simulink model "parkingNavigation_ErrorModel"  (R2021b)
settings: Solver=VariableStepAuto  StartTime=0.0  StopTime=1000  FixedStep=0.01  RelTol=1e-3
model workspace (MAT data in the model file):
  enableTransmit = 1
values from neighbouring files (symbols this model uses):
  accel_noise_deviation = 1e-3    (= 0.001)    [init.m]
  accel_scale_factor = 3e-6    (= 3e-06)    [init.m]
  accel_zero_offset = 5e-3    (= 0.005)    [init.m]
  alt_error_deviation = 1.5    [init.m]
  gyro_drift_const = deg2rad(0.02)/3600    [init.m]
  gyro_noise_deviation = deg2rad(0.01)/3600    [init.m]
  gyro_scale_factor = 5e-5    (= 5e-05)    [init.m]
  lat_error_deviation = 1.5    [init.m]
  lon_error_deviation = 1.5    [init.m]
  vel_e_error_deviation = 0.01    [init.m]
  vel_h_error_deviation = 0.01    [init.m]
  vel_n_error_deviation = 0.01    [init.m]
libraries: simulink x2
settings Model: Creator=Vladik  LastModifiedBy=Vladik

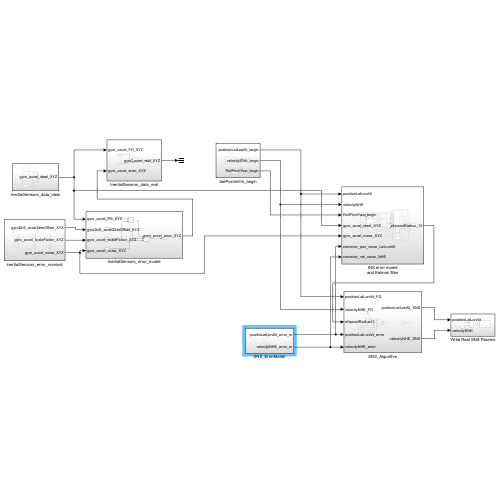
[thumbnail: Simulink's stored preview of the top-level diagram]
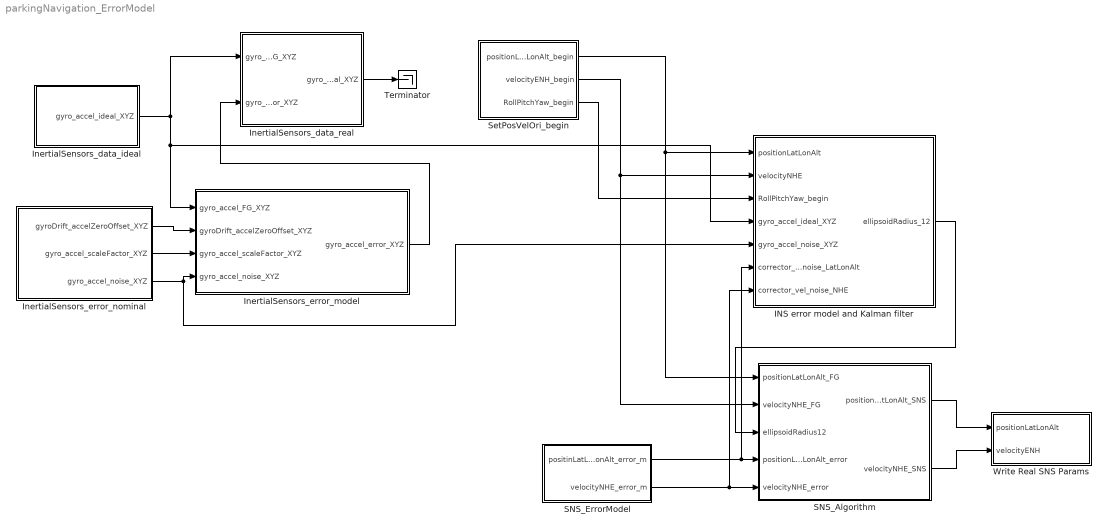
== system parkingNavigation_ErrorModel ==
  INS error model and Kalman filter : Subsystem
  InertialSensors_data_ideal : Subsystem
  InertialSensors_data_real : Subsystem
  InertialSensors_error_model : Subsystem
  InertialSensors_error_nominal : Subsystem
  SNS_Algorithm : Subsystem
  SNS_ErrorModel : Subsystem
  SetPosVelOri_begin : Subsystem
  Terminator : Terminator
  Write Real SNS Params : Subsystem
  wires:
  InertialSensors_data_ideal/1(gyro_accel_ideal_XYZ) -> InertialSensors_error_model/1(gyro_accel_FG_XYZ), INS error model and Kalman filter/4(gyro_accel_ideal_XYZ), InertialSensors_data_real/1(gyro_accel_FG_XYZ)
  InertialSensors_error_nominal/3(gyro_accel_noise_XYZ) -> InertialSensors_error_model/4(gyro_accel_noise_XYZ), INS error model and Kalman filter/5(gyro_accel_noise_XYZ)
  InertialSensors_error_nominal/2(gyro_accel_scaleFactor_XYZ) -> InertialSensors_error_model/3(gyro_accel_scaleFactor_XYZ)
  InertialSensors_error_nominal/1(gyroDrift_accelZeroOffset_XYZ) -> InertialSensors_error_model/2(gyroDrift_accelZeroOffset_XYZ)
  InertialSensors_error_model/1(gyro_accel_error_XYZ) -> InertialSensors_data_real/2(gyro_accel_error_XYZ)
  InertialSensors_data_real/1(gyro_accel_real_XYZ) -> Terminator/1
  SNS_ErrorModel/1(positinLatLonAlt_error_m) -> INS error model and Kalman filter/6(corrector_pos_noise_LatLonAlt), SNS_Algorithm/4(positionLatLonAlt_error)
  SNS_ErrorModel/2(velocityNHE_error_m) -> INS error model and Kalman filter/7(corrector_vel_noise_NHE), SNS_Algorithm/5(velocityNHE_error)
  SNS_Algorithm/1(positionLatLonAlt_SNS) -> Write Real SNS Params/1(positionLatLonAlt)
  SNS_Algorithm/2(velocityNHE_SNS) -> Write Real SNS Params/2(velocityENH)
  SetPosVelOri_begin/1(positionLatLonAlt_begin) -> INS error model and Kalman filter/1(positionLatLonAlt), SNS_Algorithm/1(positionLatLonAlt_FG)
  SetPosVelOri_begin/2(velocityENH_begin) -> INS error model and Kalman filter/2(velocityNHE), SNS_Algorithm/2(velocityNHE_FG)
  SetPosVelOri_begin/3(RollPitchYaw_begin) -> INS error model and Kalman filter/3(RollPitchYaw_begin)
  INS error model and Kalman filter/1(ellipsoidRadius_12) -> SNS_Algorithm/3(ellipsoidRadius12)

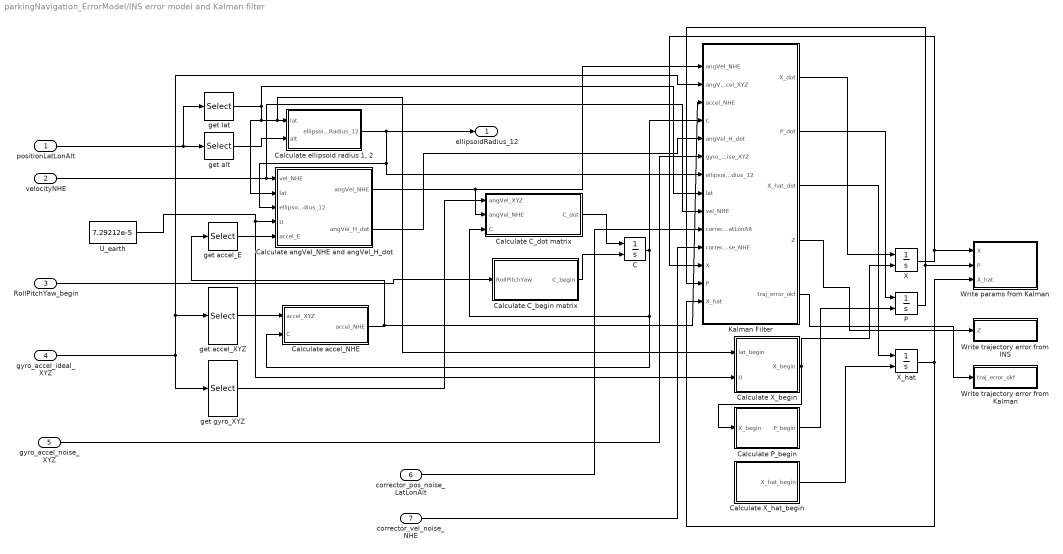
== system parkingNavigation_ErrorModel/INS error model and Kalman filter ==
  positionLatLonAlt : Inport
  velocityNHE : Inport  Port=2
  RollPitchYaw_begin : Inport  Port=3
  gyro_accel_ideal_XYZ : Inport  Port=4
  gyro_accel_noise_XYZ : Inport  Port=5
  corrector_pos_noise_LatLonAlt : Inport  Port=6
  corrector_vel_noise_NHE : Inport  Port=7
  C : Integrator  InitialConditionSource=external
  Calculate C_begin matrix : MATLAB Function  TreatAsAtomicUnit=on
  Calculate C_dot matrix : MATLAB Function  TreatAsAtomicUnit=on
  Calculate P_begin : MATLAB Function  TreatAsAtomicUnit=on
  Calculate X_begin : MATLAB Function  TreatAsAtomicUnit=on
  Calculate X_hat_begin : MATLAB Function  TreatAsAtomicUnit=on
  Calculate accel_NHE : MATLAB Function  TreatAsAtomicUnit=on
  Calculate angVel_NHE and angVel_H_dot : MATLAB Function  TreatAsAtomicUnit=on
  "Calculate ellipsoid radius 1, 2" : MATLAB Function  TreatAsAtomicUnit=on
  Kalman Filter : MATLAB Function  TreatAsAtomicUnit=on
  P : Integrator  InitialConditionSource=external
  U_earth : Constant  Value=7.29212e-5
  Write params from Kalman : Subsystem
  Write trajectory error from INS : Subsystem
  Write trajectory error from Kalman : Subsystem
  X : Integrator  InitialConditionSource=external
  X_hat : Integrator  InitialConditionSource=external
  get accel_E : Selector  InputPortWidth=3  IndexOptions=Index vector (dialog)  Indices=[3]  OutputSizes=1
  get accel_XYZ : Selector  InputPortWidth=6  IndexOptions=Index vector (dialog)  Indices=[4 5 6]  OutputSizes=1
  get alt : Selector  InputPortWidth=3  IndexOptions=Index vector (dialog)  Indices=[3]  OutputSizes=1
  get gyro_XYZ : Selector  InputPortWidth=6  IndexOptions=Index vector (dialog)  Indices=[1 2 3]  OutputSizes=1
  get lat : Selector  InputPortWidth=3  IndexOptions=Index vector (dialog)  Indices=[1]  OutputSizes=1
  ellipsoidRadius_12 : Outport
  wires:
  Kalman Filter/5(traj_error_okf) -> Write trajectory error from Kalman/1(traj_error_okf)
  corrector_vel_noise_NHE/1 -> Kalman Filter/11(corrector_vel_noise_NHE)
  gyro_accel_ideal_XYZ/1 -> get accel_XYZ/1, Kalman Filter/2(angVel_accel_XYZ), get gyro_XYZ/1
  get accel_XYZ/1 -> Calculate accel_NHE/1(accel_XYZ)
  get lat/1 -> Calculate angVel_NHE and angVel_H_dot/2(lat), Calculate X_begin/1(lat_begin), "Calculate ellipsoid radius 1, 2"/1(lat), Kalman Filter/8(lat)
  X/1 -> Write params from Kalman/1(X), Kalman Filter/12(X)
  Calculate C_begin matrix/1(C_begin) -> C/2
  C/1 -> Calculate accel_NHE/2(C), Calculate C_dot matrix/3(C), Kalman Filter/4(C)
  Calculate P_begin/1(P_begin) -> P/2
  Calculate X_hat_begin/1(X_hat_begin) -> X_hat/2
  Calculate C_dot matrix/1(C_dot) -> C/1
  X_hat/1 -> Kalman Filter/14(X_hat), Write params from Kalman/3(X_hat)
  Kalman Filter/1(X_dot) -> X/1
  gyro_accel_noise_XYZ/1 -> Kalman Filter/6(gyro_accel_noise_XYZ)
  P/1 -> Write params from Kalman/2(P), Kalman Filter/13(P)
  Calculate accel_NHE/1(accel_NHE) -> get accel_E/1, Kalman Filter/3(accel_NHE)
  Kalman Filter/2(P_dot) -> P/1
  Kalman Filter/3(X_hat_dot) -> X_hat/1
  U_earth/1 -> Calculate angVel_NHE and angVel_H_dot/4(U), Calculate X_begin/2(U)
  velocityNHE/1 -> Kalman Filter/9(vel_NHE), Calculate angVel_NHE and angVel_H_dot/1(vel_NHE)
  RollPitchYaw_begin/1 -> Calculate C_begin matrix/1(RollPitchYaw)
  Calculate angVel_NHE and angVel_H_dot/2(angVel_H_dot) -> Kalman Filter/5(angVel_H_dot)
  corrector_pos_noise_LatLonAlt/1 -> Kalman Filter/10(corrector_pos_noise_LatLonAlt)
  get accel_E/1 -> Calculate angVel_NHE and angVel_H_dot/5(accel_E)
  get gyro_XYZ/1 -> Calculate C_dot matrix/1(angVel_XYZ)
  get alt/1 -> "Calculate ellipsoid radius 1, 2"/2(alt)
  positionLatLonAlt/1 -> get lat/1, get alt/1
  Calculate angVel_NHE and angVel_H_dot/1(angVel_NHE) -> Calculate C_dot matrix/2(angVel_NHE), Kalman Filter/1(angVel_NHE)
  "Calculate ellipsoid radius 1, 2"/1(ellipsoidRadius_12) -> ellipsoidRadius_12/1, Calculate angVel_NHE and angVel_H_dot/3(ellipsoidRadius_12), Kalman Filter/7(ellipsoidRadius_12)
  Kalman Filter/4(Z) -> Write trajectory error from INS/1(Z)
  Calculate X_begin/1(X_begin) -> Calculate P_begin/1(X_begin), X/2

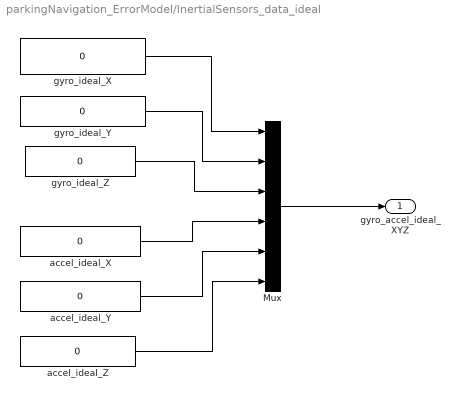
== system parkingNavigation_ErrorModel/InertialSensors_data_ideal ==
  Mux : Mux  Inputs=6
  accel_ideal_X : Constant  Value=0
  accel_ideal_Y : Constant  Value=0
  accel_ideal_Z : Constant  Value=0
  gyro_ideal_X : Constant  Value=0
  gyro_ideal_Y : Constant  Value=0
  gyro_ideal_Z : Constant  Value=0
  gyro_accel_ideal_XYZ : Outport
  wires:
  gyro_ideal_X/1 -> Mux/1
  gyro_ideal_Y/1 -> Mux/2
  gyro_ideal_Z/1 -> Mux/3
  accel_ideal_X/1 -> Mux/4
  accel_ideal_Y/1 -> Mux/5
  accel_ideal_Z/1 -> Mux/6
  Mux/1 -> gyro_accel_ideal_XYZ/1

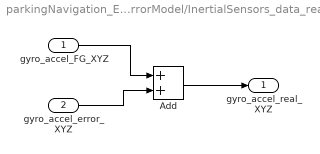
== system parkingNavigation_ErrorModel/InertialSensors_data_real ==
  gyro_accel_FG_XYZ : Inport
  gyro_accel_error_XYZ : Inport  Port=2
  Add : Sum
  gyro_accel_real_XYZ : Outport
  wires:
  Add/1 -> gyro_accel_real_XYZ/1
  gyro_accel_FG_XYZ/1 -> Add/1
  gyro_accel_error_XYZ/1 -> Add/2

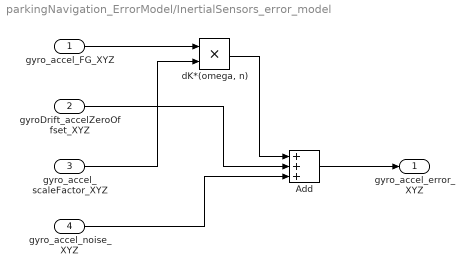
== system parkingNavigation_ErrorModel/InertialSensors_error_model ==
  gyro_accel_FG_XYZ : Inport
  gyroDrift_accelZeroOffset_XYZ : Inport  Port=2
  gyro_accel_scaleFactor_XYZ : Inport  Port=3
  gyro_accel_noise_XYZ : Inport  Port=4
  Add : Sum  Inputs=+++
  "dK*(omega, n)" : Product
  gyro_accel_error_XYZ : Outport
  wires:
  gyro_accel_scaleFactor_XYZ/1 -> "dK*(omega, n)"/2
  "dK*(omega, n)"/1 -> Add/1
  Add/1 -> gyro_accel_error_XYZ/1
  gyroDrift_accelZeroOffset_XYZ/1 -> Add/2
  gyro_accel_FG_XYZ/1 -> "dK*(omega, n)"/1
  gyro_accel_noise_XYZ/1 -> Add/3

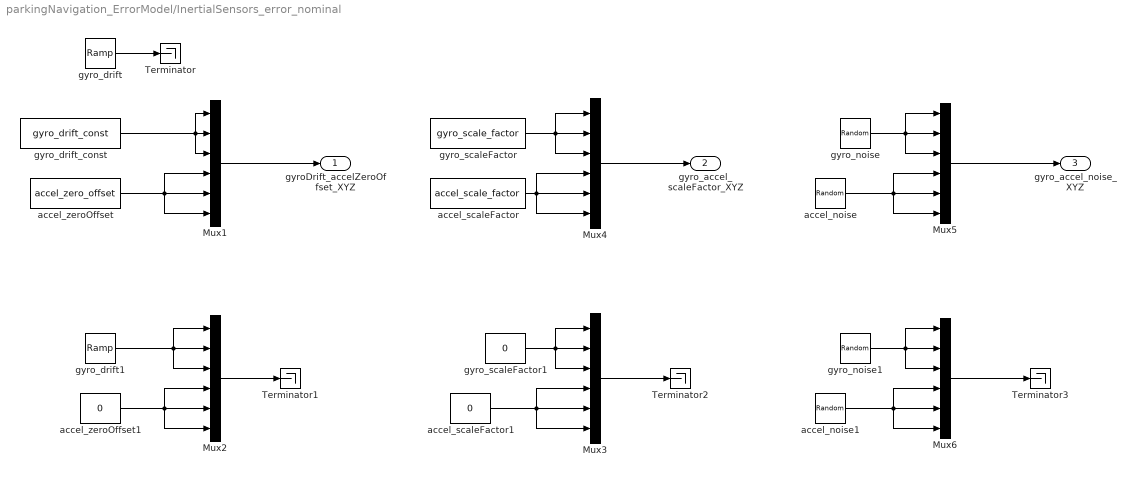
== system parkingNavigation_ErrorModel/InertialSensors_error_nominal ==
  Mux{1..6} (6 alike) : Mux  Inputs=6
  Terminator{,1..3} (4 alike) : Terminator
  accel_noise : RandomNumber  Variance=accel_noise_deviation^2  SampleTime=1
  accel_noise1 : RandomNumber  Variance=0  SampleTime=1
  accel_scaleFactor : Constant  Value=accel_scale_factor
  accel_scaleFactor1 : Constant  Value=0
  accel_zeroOffset : Constant  Value=accel_zero_offset  VectorParams1D=off
  accel_zeroOffset1 : Constant  Value=0
  gyro_drift : simulink/Sources/Ramp  slope=0.015*pi/180/3600  start=0  InitialOutput=0
  gyro_drift1 : simulink/Sources/Ramp  slope=0  start=0  InitialOutput=0
  gyro_drift_const : Constant  Value=gyro_drift_const
  gyro_noise : RandomNumber  Variance=gyro_noise_deviation^2  SampleTime=1
  gyro_noise1 : RandomNumber  Variance=0  SampleTime=1
  gyro_scaleFactor : Constant  Value=gyro_scale_factor
  gyro_scaleFactor1 : Constant  Value=0
  gyroDrift_accelZeroOffset_XYZ : Outport
  gyro_accel_scaleFactor_XYZ : Outport  Port=2
  gyro_accel_noise_XYZ : Outport  Port=3
  wires:
  accel_noise/1 -> Mux5/6, Mux5/5, Mux5/4
  accel_scaleFactor/1 -> Mux4/6, Mux4/5, Mux4/4
  Mux5/1 -> gyro_accel_noise_XYZ/1
  Mux4/1 -> gyro_accel_scaleFactor_XYZ/1
  Mux1/1 -> gyroDrift_accelZeroOffset_XYZ/1
  accel_zeroOffset/1 -> Mux1/5, Mux1/6, Mux1/4
  gyro_scaleFactor/1 -> Mux4/3, Mux4/2, Mux4/1
  gyro_noise/1 -> Mux5/3, Mux5/2, Mux5/1
  accel_zeroOffset1/1 -> Mux2/5, Mux2/6, Mux2/4
  gyro_noise1/1 -> Mux6/3, Mux6/2, Mux6/1
  gyro_scaleFactor1/1 -> Mux3/3, Mux3/2, Mux3/1
  gyro_drift1/1 -> Mux2/3, Mux2/1, Mux2/2
  accel_noise1/1 -> Mux6/6, Mux6/5, Mux6/4
  accel_scaleFactor1/1 -> Mux3/6, Mux3/5, Mux3/4
  gyro_drift_const/1 -> Mux1/1, Mux1/2, Mux1/3
  gyro_drift/1 -> Terminator/1
  Mux2/1 -> Terminator1/1
  Mux3/1 -> Terminator2/1
  Mux6/1 -> Terminator3/1

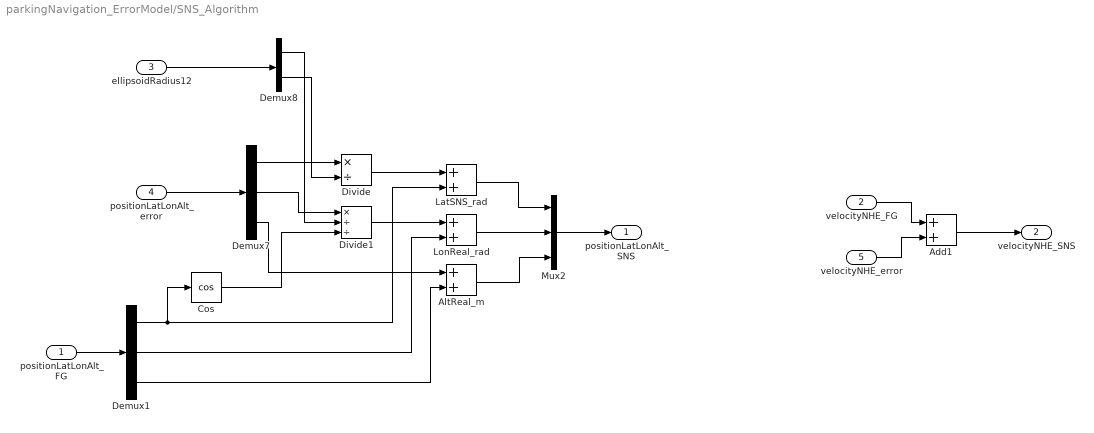
== system parkingNavigation_ErrorModel/SNS_Algorithm ==
  positionLatLonAlt_FG : Inport
  velocityNHE_FG : Inport  Port=2
  ellipsoidRadius12 : Inport  Port=3
  positionLatLonAlt_error : Inport  Port=4
  velocityNHE_error : Inport  Port=5
  Add1 : Sum
  AltReal_m : Sum
  Cos : Trigonometry  Operator=cos
  Demux1 : Demux  Outputs=3
  Demux7 : Demux  Outputs=3
  Demux8 : Demux  Outputs=2
  Divide : Product  Inputs=*/
  Divide1 : Product  Inputs=*//
  LatSNS_rad : Sum
  LonReal_rad : Sum
  Mux2 : Mux  Inputs=3
  positionLatLonAlt_SNS : Outport
  velocityNHE_SNS : Outport  Port=2
  wires:
  Divide1/1 -> LonReal_rad/1
  Divide/1 -> LatSNS_rad/1
  ellipsoidRadius12/1 -> Demux8/1
  positionLatLonAlt_error/1 -> Demux7/1
  Demux7/1 -> Divide/1
  Demux7/2 -> Divide1/1
  Demux1/1 -> LatSNS_rad/2, Cos/1
  Cos/1 -> Divide1/3
  positionLatLonAlt_FG/1 -> Demux1/1
  Demux1/2 -> LonReal_rad/2
  Demux7/3 -> AltReal_m/1
  Demux1/3 -> AltReal_m/2
  LonReal_rad/1 -> Mux2/2
  LatSNS_rad/1 -> Mux2/1
  AltReal_m/1 -> Mux2/3
  Mux2/1 -> positionLatLonAlt_SNS/1
  velocityNHE_FG/1 -> Add1/1
  velocityNHE_error/1 -> Add1/2
  Add1/1 -> velocityNHE_SNS/1
  Demux8/2 -> Divide/2
  Demux8/1 -> Divide1/2

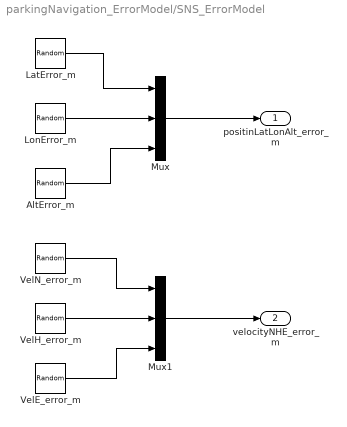
== system parkingNavigation_ErrorModel/SNS_ErrorModel ==
  AltError_m : RandomNumber  Variance=alt_error_deviation^2  Seed=1  SampleTime=0.1
  LatError_m : RandomNumber  Variance=lat_error_deviation^2  Seed=1  SampleTime=0.1
  LonError_m : RandomNumber  Variance=lon_error_deviation^2  Seed=1  SampleTime=0.1
  Mux : Mux  Inputs=3
  Mux1 : Mux  Inputs=3
  VelE_error_m : RandomNumber  Variance=vel_e_error_deviation^2  Seed=2  SampleTime=0.1
  VelH_error_m : RandomNumber  Variance=vel_h_error_deviation^2  Seed=2  SampleTime=0.1
  VelN_error_m : RandomNumber  Variance=vel_n_error_deviation^2  Seed=2  SampleTime=0.1
  positinLatLonAlt_error_m : Outport
  velocityNHE_error_m : Outport  Port=2
  wires:
  LonError_m/1 -> Mux/2
  LatError_m/1 -> Mux/1
  AltError_m/1 -> Mux/3
  Mux/1 -> positinLatLonAlt_error_m/1
  Mux1/1 -> velocityNHE_error_m/1
  VelH_error_m/1 -> Mux1/2
  VelN_error_m/1 -> Mux1/1
  VelE_error_m/1 -> Mux1/3

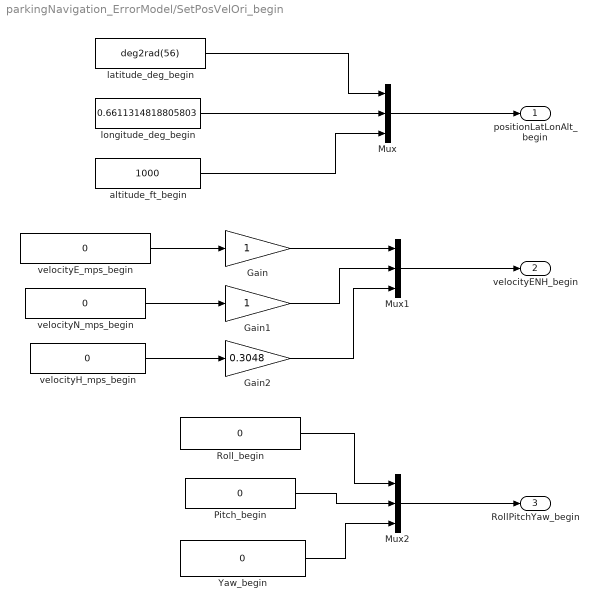
== system parkingNavigation_ErrorModel/SetPosVelOri_begin ==
  Gain : Gain
  Gain1 : Gain
  Gain2 : Gain  Gain=0.3048
  Mux : Mux  Inputs=3
  Mux1 : Mux  Inputs=3
  Mux2 : Mux  Inputs=3
  Pitch_begin : Constant  Value=0
  Roll_begin : Constant  Value=0
  Yaw_begin : Constant  Value=0
  altitude_ft_begin : Constant  Value=1000
  latitude_deg_begin : Constant  Value=deg2rad(56)
  longitude_deg_begin : Constant  Value=0.6611314818805803
  velocityE_mps_begin : Constant  Value=0
  velocityH_mps_begin : Constant  Value=0
  velocityN_mps_begin : Constant  Value=0
  positionLatLonAlt_begin : Outport
  velocityENH_begin : Outport  Port=2
  RollPitchYaw_begin : Outport  Port=3
  wires:
  Mux1/1 -> velocityENH_begin/1
  longitude_deg_begin/1 -> Mux/2
  altitude_ft_begin/1 -> Mux/3
  latitude_deg_begin/1 -> Mux/1
  Mux/1 -> positionLatLonAlt_begin/1
  Yaw_begin/1 -> Mux2/3
  Pitch_begin/1 -> Mux2/2
  Roll_begin/1 -> Mux2/1
  Mux2/1 -> RollPitchYaw_begin/1
  Gain/1 -> Mux1/1
  velocityE_mps_begin/1 -> Gain/1
  velocityN_mps_begin/1 -> Gain1/1
  Gain1/1 -> Mux1/2
  velocityH_mps_begin/1 -> Gain2/1
  Gain2/1 -> Mux1/3

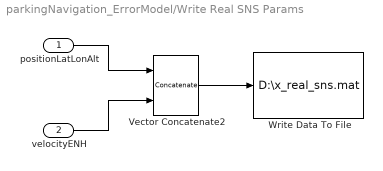
== system parkingNavigation_ErrorModel/Write Real SNS Params ==
  positionLatLonAlt : Inport
  velocityENH : Inport  Port=2
  Vector Concatenate2 : Concatenate  Mode=Multidimensional array
  Write Data To File : ToFile  Filename=D:\x_real_sns.mat  MatrixName=x_real_sns
  wires:
  positionLatLonAlt/1 -> Vector Concatenate2/1
  Vector Concatenate2/1 -> Write Data To File/1
  velocityENH/1 -> Vector Concatenate2/2

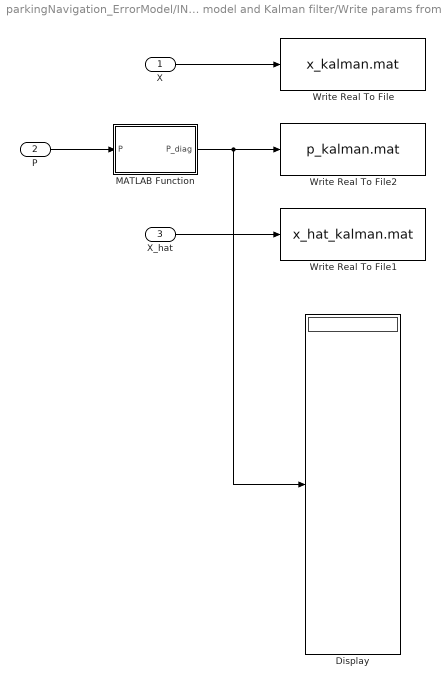
== system parkingNavigation_ErrorModel/INS error model and Kalman filter/Write params from Kalman ==
  X : Inport
  P : Inport  Port=2
  X_hat : Inport  Port=3
  Display : Display
  MATLAB Function : MATLAB Function  TreatAsAtomicUnit=on
  Write Real To File : ToFile  Filename=x_kalman.mat  MatrixName=x_kalman
  Write Real To File1 : ToFile  Filename=x_hat_kalman.mat  MatrixName=x_hat_kalman
  Write Real To File2 : ToFile  Filename=p_kalman.mat  MatrixName=p_kalman
  wires:
  X/1 -> Write Real To File/1
  X_hat/1 -> Write Real To File1/1
  MATLAB Function/1(P_diag) -> Display/1, Write Real To File2/1
  P/1 -> MATLAB Function/1(P)

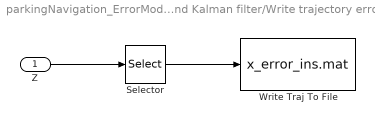
== system parkingNavigation_ErrorModel/INS error model and Kalman filter/Write trajectory error from INS ==
  Z : Inport
  Selector : Selector  InputPortWidth=4  IndexOptions=Index vector (dialog)  Indices=[1 2]  OutputSizes=1
  Write Traj To File : ToFile  Filename=x_error_ins.mat  MatrixName=x_error_ins
  wires:
  Z/1 -> Selector/1
  Selector/1 -> Write Traj To File/1

== system parkingNavigation_ErrorModel/INS error model and Kalman filter/Write trajectory error from Kalman ==
  traj_error_okf : Inport
  Write Traj To File : ToFile  Filename=x_error_okf.mat  MatrixName=x_error_okf
  wires:
  traj_error_okf/1 -> Write Traj To File/1

== matlab function parkingNavigation_ErrorModel/INS error model and Kalman filter/Calculate X_begin ==
  data: X_begin output; lat_begin input; U input
function X_begin = fcn(lat_begin, U)

    x1_begin = 20;
    x2_begin = 20;
    d_vel_E = 1;
    d_vel_N = 1;
    alpha_begin = deg2rad(0.02);
    beta_begin = deg2rad(0.02);
    gamma_begin = deg2rad(0.02);
    %gyro_drift_begin = 0.015*pi/180/3600;
    gyro_drift_begin = deg2rad(0.015) / 3600;
    %gyro_scaleFactor_begin = 5e-4;
    gyro_scaleFactor_begin = 5e-4;
    %accel_zeroOffset_begin = 5e-4;
    accel_zeroOffset_begin = 5e-4;
    %accel_scaleFactor_begin = 3e-5;
    accel_scaleFactor_begin = 3e-5;

    x3_begin = d_vel_E + U * sin(lat_begin) * x2_begin;
    x4_begin = d_vel_N;

    X_begin = [x1_begin, x2_begin, x3_begin, x4_begin, alpha_begin, beta_begin, gamma_begin, ...
        gyro_drift_begin, gyro_drift_begin, gyro_drift_begin, ...
        gyro_scaleFactor_begin, gyro_scaleFactor_begin, gyro_scaleFactor_begin, ...
        accel_zeroOffset_begin, accel_zeroOffset_begin, accel_zeroOffset_begin, ...
        accel_scaleFactor_begin, accel_scaleFactor_begin, accel_scaleFactor_begin]';
end

== matlab function parkingNavigation_ErrorModel/INS error model and Kalman filter/Calculate X_hat_begin ==
  data: X_hat_begin output
function X_hat_begin = fcn()

    X_hat_begin = zeros(19, 1);

end

== matlab function parkingNavigation_ErrorModel/INS error model and Kalman filter/Calculate P_begin ==
  data: P_begin output; X_begin input
function P_begin = fcn(X_begin)

    %P_begin = diag(X_begin).^2;
    P_begin = X_begin * X_begin';

end

== matlab function parkingNavigation_ErrorModel/INS error model and Kalman filter/Write params from Kalman/MATLAB Function ==
  data: P input; P_diag output
function P_diag = get_diag(P)
    P_diag = zeros(19, 1);
    for i = 1:1:19
        P_diag(i) = P(i, i);
    end
end

== matlab function parkingNavigation_ErrorModel/INS error model and Kalman filter/Calculate ellipsoid radius 1, 2 ==
  data: lat input; ellipsoidRadius_12 output; alt input
function ellipsoidRadius_12 = fcn(lat, alt)
    
    a = 6378245; %big semiaxis
    b = 6356863; %small semiaxis
    e = (a^2 - b^2) / a^2; %square of the first eccentricity
    denom = sqrt(1 - e^2 * sin(lat)^2); %denominator

    ro1 = a * (1 - e^2) / denom^3 + alt;
    ro2 = a / denom + alt;
    ellipsoidRadius_12 = [ro1; ro2];
end

== matlab function parkingNavigation_ErrorModel/INS error model and Kalman filter/Kalman Filter ==
  data: X_dot output; angVel_NHE input; angVel_accel_XYZ input; accel_NHE input; C input; angVel_H_dot input; gyro_accel_noise_XYZ input; ellipsoidRadius_12 input; lat input; vel_NHE input; corrector_pos_noise_LatLonAlt input; corrector_vel_noise_NHE input; X input; P input; X_hat input; P_dot output; X_hat_dot output; Z output; traj_error_okf output
function [X_dot, P_dot, X_hat_dot, Z, traj_error_okf] = fcn(angVel_NHE, angVel_accel_XYZ, accel_NHE, C, angVel_H_dot, gyro_accel_noise_XYZ, ellipsoidRadius_12, lat, vel_NHE, corrector_pos_noise_LatLonAlt, corrector_vel_noise_NHE, X, P, X_hat)

omega_0 = 1.25e-3;

    angVel_E = angVel_NHE(3);
    angVel_N = angVel_NHE(1);
    angVel_H = angVel_NHE(2);
    angVel_X = angVel_accel_XYZ(1);
    angVel_Y = angVel_accel_XYZ(2);
    angVel_Z = angVel_accel_XYZ(3);
    accel_E = accel_NHE(3);
    accel_N = accel_NHE(1);
    accel_H = accel_NHE(2);
    accel_X = angVel_accel_XYZ(4);
    accel_Y = angVel_accel_XYZ(5);
    accel_Z = angVel_accel_XYZ(6);
    gyroNoise_X = gyro_accel_noise_XYZ(1);
    gyroNoise_Y = gyro_accel_noise_XYZ(2);
    gyroNoise_Z = gyro_accel_noise_XYZ(3);
    accelNoise_X = gyro_accel_noise_XYZ(4);
    accelNoise_Y = gyro_accel_noise_XYZ(5);
    accelNoise_Z = gyro_accel_noise_XYZ(6);
    ro_1 = ellipsoidRadius_12(1);
    ro_2 = ellipsoidRadius_12(2);
    %vel_N = vel_NHE(1);
    vel_H = vel_NHE(2);
    %vel_E = vel_NHE(3);
    corrector_pos_noise_lat = corrector_pos_noise_LatLonAlt(1);
    corrector_pos_noise_lon = corrector_pos_noise_LatLonAlt(2);
    %corrector_pos_noise_alt = corrector_pos_noise_LatLonAlt(3);
    corrector_vel_noise_N = corrector_vel_noise_NHE(1);
    %corrector_vel_noise_H = corrector_vel_noise_NHE(2);
    corrector_vel_noise_E = corrector_vel_noise_NHE(3);

    F = zeros(19, 19);
    G = zeros(19, 6);
    H = zeros(4, 19);

    %create system state matrix F
    F(1, 3) = 1;
    F(2, 4) = 1;
    F(3, :) = [-omega_0^2 + angVel_N^2 + angVel_H^2, angVel_H_dot - angVel_E * angVel_N, 0, 2 * angVel_H, 0, accel_H, -accel_N, 0, 0, 0, 0, 0, 0, C(1,1), C(1,2), C(1,3), accel_X * C(1, 1), accel_Y * C(1, 2), accel_Z * C(1, 3)];
    F(4, :) = [-(angVel_H_dot - angVel_E * angVel_N), -omega_0^2 + angVel_E^2 + angVel_H^2, -2 * angVel_H, 0, accel_H, 0, -accel_E, 0, 0, 0, 0, 0, 0, C(2,1), C(2,2), C(2,3), accel_X * C(2, 1), accel_Y * C(2, 2), accel_Z * C(2, 3)];
    F(5, :) = [0, 0, 0, 0, 0, angVel_H, -angVel_N, C(1,1), C(1,2), C(1,3), angVel_X * C(1, 1), angVel_Y * C(1, 2), angVel_Z * C(1, 3), 0, 0, 0, 0, 0, 0];
    F(6, :) = [0, 0, 0, 0, -angVel_H, 0, angVel_E, C(2,1), C(2,2), C(2,3), angVel_X * C(2, 1), angVel_Y * C(2, 2), angVel_Z * C(2, 3), 0, 0, 0, 0, 0, 0];
    F(7, :) = [0, 0, 0, 0, angVel_N, -angVel_E, 0, C(3,1), C(3,2), C(3,3), angVel_X * C(3, 1), angVel_Y * C(3, 2), angVel_Z * C(3, 3), 0, 0, 0, 0, 0, 0];

    %create system noise matrix G
    G(3, :) = [0, 0, 0, C(1,1), C(1,2), C(1,3)];
    G(4, :) = [0, 0, 0, C(2,1), C(2,2), C(2,3)];
    G(5, :) = [C(1,1), C(1,2), C(1,3), 0, 0, 0];
    G(6, :) = [C(2,1), C(2,2), C(2,3), 0, 0, 0];
    G(7, :) = [C(3,1), C(3,2), C(3,3), 0, 0, 0];
    
    %create noise vectors W and V
    W = [gyroNoise_X, gyroNoise_Y, gyroNoise_Z, accelNoise_X, accelNoise_Y, accelNoise_Z]';
    V = [corrector_pos_noise_lat, corrector_pos_noise_lon, corrector_vel_noise_E, corrector_vel_noise_N]';

    X_dot = F * X + G * W;

    %create measurement matrix H
    H(1, 1) = 1 / (ro_2 * cos(lat));
    H(2, 2) = 1 / ro_1;
    H(3, 1) = -(vel_H / ro_2 + angVel_E * tan(lat));
    H(3, 2) = -angVel_H;
    H(3, 3) = 1;
    H(4, 1) = -vel_H / ro_1;
    H(4, 4) = 1;

    Y = H * X;
    Z = Y + V;

    lat_error_hat = X_hat(1) / (ro_2 * cos(lat));
    lon_error_hat = X_hat(2) / ro_1;
    traj_error_okf = [lat_error_hat, lon_error_hat]';

    SNS_errors = [1.5, 1.5, 0.01, 0.01]';
    R = diag(SNS_errors).^2;
    R_inv = inv(R);

    inertial_sensors_error = [deg2rad(0.01)/3600, deg2rad(0.01)/3600, deg2rad(0.01)/3600, ...
        1e-3, 1e-3, 1e-3]';
    Q = diag(inertial_sensors_error).^2;

    P_dot = F * P + P * F' - P * H' * R_inv * H * P + G * Q * G';
    K = P * H' * R_inv;
    X_hat_dot = F * X_hat + K * (Z - H * X_hat);

== matlab function parkingNavigation_ErrorModel/INS error model and Kalman filter/Calculate angVel_NHE and angVel_H_dot ==
  data: vel_NHE input; lat input; angVel_NHE output; ellipsoidRadius_12 input; U input; accel_E input; angVel_H_dot output
function [angVel_NHE, angVel_H_dot] = fcn(vel_NHE, lat, ellipsoidRadius_12, U, accel_E)
    angVel_E = -vel_NHE(1) / ellipsoidRadius_12(1);
    angVel_N = vel_NHE(3) / ellipsoidRadius_12(2) + U * cos(lat);
    angVel_H = vel_NHE(3) / ellipsoidRadius_12(2) * tan(lat) + U * sin(lat);
    
    angVel_NHE = [angVel_N; angVel_H; angVel_E];

    angVel_H_dot = (U * cos(lat) * vel_NHE(1) + accel_E * tan(lat) + vel_NHE(2) * angVel_NHE(2) + vel_NHE(3) * vel_NHE(1) / ...
        (ellipsoidRadius_12(2) * cos(lat)^2)) / ellipsoidRadius_12(2);

end

== matlab function parkingNavigation_ErrorModel/INS error model and Kalman filter/Calculate accel_NHE ==
  data: accel_XYZ input; accel_NHE output; C input
function accel_NHE = fcn(accel_XYZ, C)
    
    accel_NHE = C * accel_XYZ;
end

== matlab function parkingNavigation_ErrorModel/INS error model and Kalman filter/Calculate C_dot matrix ==
  data: C_dot output; angVel_XYZ input; angVel_NHE input; C input
function C_dot = fcn(angVel_XYZ, angVel_NHE, C)
    
    angVel_XYZ_matrix = [ 0, -angVel_XYZ(3), angVel_XYZ(2);
                        angVel_XYZ(3), 0, -angVel_XYZ(1);
                        -angVel_XYZ(2), angVel_XYZ(1), 0 ];
    angVel_NHE_matrix = [ 0, -angVel_NHE(3), angVel_NHE(2);
                        angVel_NHE(3), 0, -angVel_NHE(1);
                        -angVel_NHE(2), angVel_NHE(1), 0 ];
    
    C_dot = C * angVel_XYZ_matrix - angVel_NHE_matrix * C;

end

== matlab function parkingNavigation_ErrorModel/INS error model and Kalman filter/Calculate C_begin matrix ==
  data: RollPitchYaw input; C_begin output
function C_begin = fcn(RollPitchYaw)
    cos_roll = cos(RollPitchYaw(1));
    cos_pitch = cos(RollPitchYaw(2));
    cos_yaw = cos(RollPitchYaw(3));
    sin_roll = sin(RollPitchYaw(1));
    sin_pitch = sin(RollPitchYaw(2));
    sin_yaw = sin(RollPitchYaw(3));

    C_begin = zeros(3, 3);
    C_begin(:, 1) = [cos_pitch * cos_yaw; %left column
                    sin_pitch;
                    -cos_pitch * sin_yaw];
    C_begin(:, 2) = [-cos_roll * cos_yaw * sin_pitch + sin_roll * sin_yaw; %middle column
                    cos_roll * cos_pitch;
                    cos_roll * sin_yaw * sin_pitch + sin_roll * cos_yaw];
    C_begin(:, 3) = [sin_roll * cos_yaw * sin_pitch + cos_roll * sin_yaw; %right column
                    -sin_roll * cos_pitch;
                    -sin_roll * sin_yaw * sin_pitch + cos_roll * cos_yaw];
end
